simulink model "joystick"  (R2020a)
settings: Solver=VariableStepAuto  StartTime=0.0  StopTime=50  RelTol=1e-3
libraries: aerolibanimutils x2
settings Model: Creator=Khojasteh Mirza  LastModifiedBy=Khojasteh Mirza

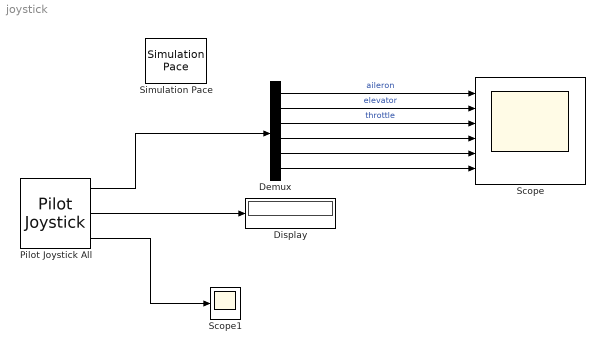
== system joystick ==
  Demux : Demux  Outputs=6
  Display : Display
  Pilot Joystick All : aerolibanimutils/Pilot Joystick  JoystickID=Joystick1  OutputConfiguration=AllOutputs  SampleTime=1/50
  Scope : Scope  NumInputPorts=6
  Scope1 : Scope
  Simulation Pace : aerolibanimutils/Simulation Pace  SimulationPace=1  SleepMode=Auto  OutputPaceError=off  SampleTime=1/50
  wires:
  Pilot Joystick All/3 -> Scope1/1
  Pilot Joystick All/2 -> Display/1
  Pilot Joystick All/1 -> Demux/1
  Demux/1 -> Scope/1  "aileron"
  Demux/2 -> Scope/2  "elevator"
  Demux/3 -> Scope/3  "throttle"
  Demux/6 -> Scope/6
  Demux/5 -> Scope/5
  Demux/4 -> Scope/4
